simulink model "RCAMSimulation"  (R2024b)
settings: Solver=VariableStepAuto  StartTime=0.0  StopTime=TF  FixedStep=0.05  RelTol=1e-3
values from neighbouring files (symbols this model uses):
  u1max = deg2rad(25)    [RCAM_model.m]    (also in RCAM_model_navigation.m)
  u1min = deg2rad(-25)    [RCAM_model.m]    (also in RCAM_model_navigation.m)
  u2max = deg2rad(10)    [RCAM_model.m]    (also in RCAM_model_navigation.m)
  u2min = deg2rad(-25)    [RCAM_model.m]    (also in RCAM_model_navigation.m)
  u3max = deg2rad(30)    [RCAM_model.m]    (also in RCAM_model_navigation.m)
  u3min = deg2rad(-30)    [RCAM_model.m]    (also in RCAM_model_navigation.m)
  u4max = deg2rad(10)    [RCAM_model.m]    (also in RCAM_model_navigation.m)
  u4min = deg2rad(0.5)    [RCAM_model.m]    (also in RCAM_model_navigation.m)
  u5max = u4max    [RCAM_model.m]    (also in RCAM_model_navigation.m)
  u5min = u4min    [RCAM_model.m]    (also in RCAM_model_navigation.m)
  U_bar = Z_bar(10:14)    [RCAM_LQR_Trim.m]    (also in RCAM_LQR_Trim_navigation.m = Z_bar(13:17))
  X_bar = Z_bar(1:9)    [RCAM_LQR_Trim.m]    (also in RCAM_LQR_Trim_navigation.m)
undefined symbols (not defined in the file or in its folder): ail_dist, dist_dt, GEO0, K, navigation_from_state, P0, RB211, RCAM_model, rud_dist, stab_dist, x0
libraries: aerolibfltsims x2, vrlib x1, aerolibanimutils x1
settings Model: Creator=jaspergeldenbott  LastModifiedBy=jaspergeldenbott
settings RTWCC: GPUComputeCapability=3.5

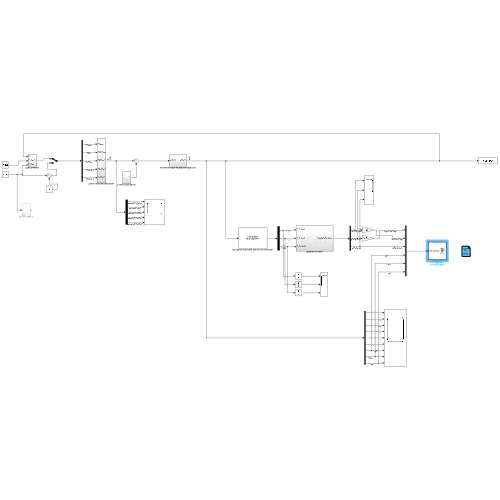
[thumbnail: Simulink's stored preview of the top-level diagram]
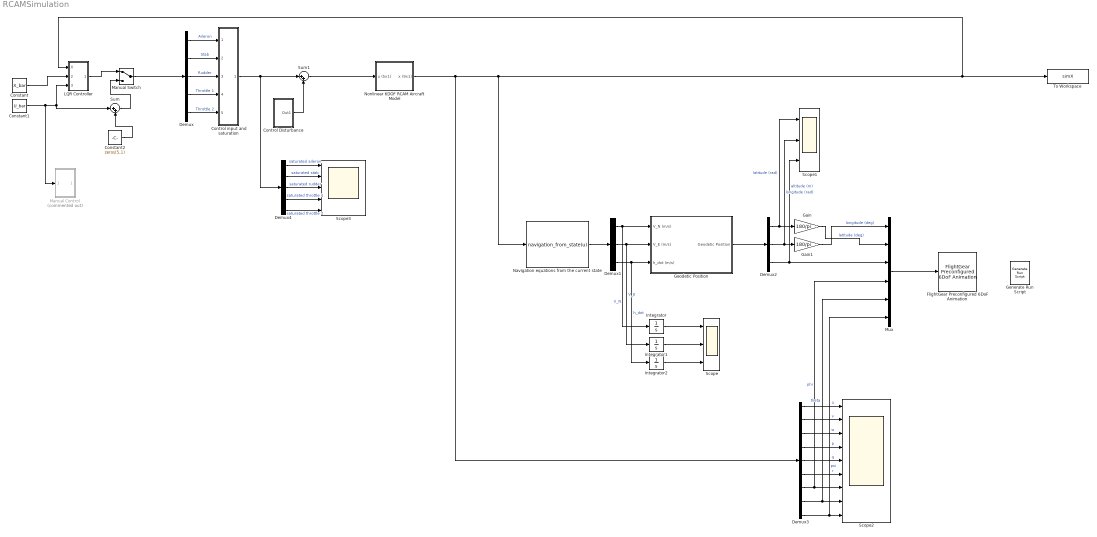
== system RCAMSimulation ==
  Constant : Constant  Value=X_bar
  Constant1 : Constant  Value=U_bar
  Constant2 : Constant  Value=zeros(5,1)
  Control Disturbance : Subsystem
  Control input and saturation : Subsystem
  Demux : Demux  Outputs=5
  Demux1 : Demux  Outputs=3
  Demux2 : Demux  Outputs=3
  Demux3 : Demux  Outputs=9
  Demux4 : Demux  Outputs=5
  FlightGear Preconfigured 6DoF Animation : aerolibfltsims/FlightGear Preconfigured 6DoF Animation  xFlightGearVersion=v2019.1  DestinationIpAddress=127.0.0.1  DestinationPort=5502  SampleTime=1/200  packetVersion=24
  Gain : Gain  Gain=180/pi
  Gain1 : Gain  Gain=180/pi
  Generate Run Script : aerolibfltsims/Generate Run Script  Architecture=Mac  dataFlow=Send  GeometryModelName=757-200-RB211  AirportId=KSFO  RunwayId=10L  InitialAltitude=7224  InitialHeading=113  OffsetDistance=4.72  OffsetAzimuth=0  InstallScenery=off  DisableShaders=off  OriginAddress=127.0.0.1  DestinationPort=5502  OriginPort=5505  LocalAddress=127.0.0.1  OutputFileName=runfg.bat  FlightGearBaseDirectory=/Applications/FlightGear.app
  Geodetic Position : Subsystem
  Integrator : Integrator  InitialCondition=P0(1)
  Integrator1 : Integrator  InitialCondition=P0(2)
  Integrator2 : Integrator  InitialCondition=P0(3)
  LQR Controller : Subsystem
  Manual Control : Subsystem  Commented=on
  Manual Switch : ManualSwitch
  Mux : Mux  Inputs=6
  Navigation equations from the current state : MATLABFcn  MATLABFcn=navigation_from_state(u)
  Nonlinear 6DOF RCAM Aircraft Model : Subsystem
  Scope : Scope  NumInputPorts=3
  Scope1 : Scope  NumInputPorts=3
  Scope2 : Scope  NumInputPorts=9
  Scope3 : Scope  NumInputPorts=5
  Sum : Sum  Inputs=|++
  Sum1 : Sum  Inputs=|++
  To Workspace : ToWorkspace  VariableName=simX  SaveFormat=Timeseries  SampleTime=-1
  wires:
  Nonlinear 6DOF RCAM Aircraft Model/1(x (9x1)) -> To Workspace/1, LQR Controller/1(X), Navigation equations from the current state/1, Demux3/1
  Demux/4 -> Control input and saturation/4(Throttle 1)  "Throttle 1"
  Demux/3 -> Control input and saturation/3(Rudder)  "Rudder"
  Demux/1 -> Control input and saturation/1(Aileron)  "Aileron"
  Demux/5 -> Control input and saturation/5(Trottle 2)  "Throttle 2"
  Demux/2 -> Control input and saturation/2(Stabilizer)  "Stab"
  Navigation equations from the current state/1 -> Demux1/1
  Demux1/1 -> Integrator/1, Geodetic Position/1(V_N (m/s))  "V_N"
  Demux1/2 -> Integrator1/1, Geodetic Position/2(V_E (m/s))  "V_E"
  Demux1/3 -> Integrator2/1, Geodetic Position/3(h_dot (m/s))  "h_dot"
  Integrator/1 -> Scope/1
  Integrator1/1 -> Scope/2
  Integrator2/1 -> Scope/3
  Geodetic Position/1(Geodetic Position) -> Demux2/1
  Demux2/1 -> Scope1/1, Gain/1  "latitude (rad)"
  Demux2/2 -> Scope1/2, Gain1/1  "longitude (rad)"
  Demux2/3 -> Scope1/3, Mux/3  "altitude (m)"
  Constant/1 -> LQR Controller/2(X_bar)
  Constant1/1 -> Manual Control/1(In1), LQR Controller/3(U_bar), Sum/1
  LQR Controller/1(Out1) -> Manual Switch/1
  Gain1/1 -> Mux/1  "longitude (deg)"
  Gain/1 -> Mux/2  "latitude (deg)"
  Mux/1 -> FlightGear Preconfigured 6DoF Animation/1
  Demux3/1 -> Scope2/1  "u"
  Demux3/2 -> Scope2/2  "v"
  Demux3/3 -> Scope2/3  "w"
  Demux3/4 -> Scope2/4  "p"
  Demux3/5 -> Scope2/5  "q"
  Demux3/6 -> Scope2/6  "r"
  Demux3/7 -> Mux/4, Scope2/7  "phi"
  Demux3/8 -> Mux/5, Scope2/8  "theta"
  Demux3/9 -> Mux/6, Scope2/9  "psi"
  Control Disturbance/1(Out1) -> Sum1/2
  Constant2/1 -> Sum/2
  Sum/1 -> Manual Switch/2
  Control input and saturation/1(Out1) -> Demux4/1, Sum1/1
  Sum1/1 -> Nonlinear 6DOF RCAM Aircraft Model/1(u (5x1))
  Manual Switch/1 -> Demux/1
  Demux4/1 -> Scope3/1  "saturated aileron"
  Demux4/2 -> Scope3/2  "saturated stab"
  Demux4/3 -> Scope3/3  "saturated rudder"
  Demux4/4 -> Scope3/4  "saturated throttle 1"
  Demux4/5 -> Scope3/5  "saturated throttle 2"

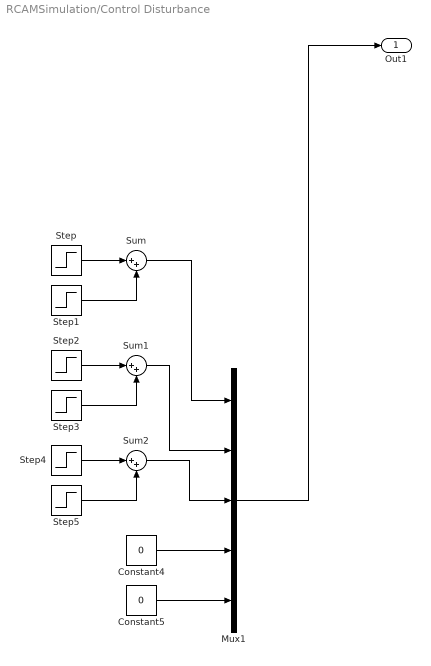
== system RCAMSimulation/Control Disturbance ==
  Constant4 : Constant  Value=0
  Constant5 : Constant  Value=0
  Mux1 : Mux  Inputs=5
  Step : Step  Time=10  After=ail_dist*pi/180  SampleTime=0
  Step1 : Step  Time=10 + dist_dt  After=-ail_dist*pi/180  SampleTime=0
  Step2 : Step  Time=10  After=stab_dist*pi/180  SampleTime=0
  Step3 : Step  Time=10 + dist_dt  After=-stab_dist*pi/180  SampleTime=0
  Step4 : Step  Time=10  After=rud_dist*pi/180  SampleTime=0
  Step5 : Step  Time=10 + dist_dt  After=-rud_dist*pi/180  SampleTime=0
  Sum : Sum  Inputs=|++
  Sum1 : Sum  Inputs=|++
  Sum2 : Sum  Inputs=|++
  Out1 : Outport
  wires:
  Sum/1 -> Mux1/1
  Constant5/1 -> Mux1/5
  Sum1/1 -> Mux1/2
  Step1/1 -> Sum/2
  Mux1/1 -> Out1/1
  Step/1 -> Sum/1
  Constant4/1 -> Mux1/4
  Step3/1 -> Sum1/2
  Step2/1 -> Sum1/1
  Step5/1 -> Sum2/2
  Step4/1 -> Sum2/1
  Sum2/1 -> Mux1/3

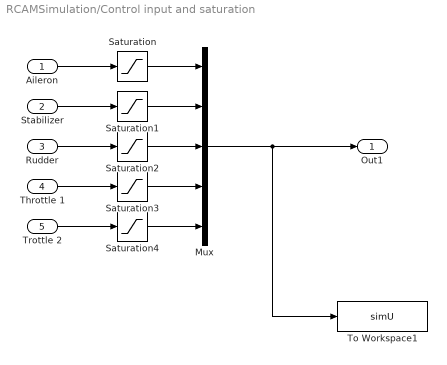
== system RCAMSimulation/Control input and saturation ==
  Aileron : Inport
  Stabilizer : Inport  Port=2
  Rudder : Inport  Port=3
  Throttle 1 : Inport  Port=4
  Trottle 2 : Inport  Port=5
  Mux : Mux  Inputs=5
  Saturation : Saturate  UpperLimit=u1max  LowerLimit=u1min
  Saturation1 : Saturate  UpperLimit=u2max  LowerLimit=u2min
  Saturation2 : Saturate  UpperLimit=u3max  LowerLimit=u3min
  Saturation3 : Saturate  UpperLimit=u4max  LowerLimit=u4min
  Saturation4 : Saturate  UpperLimit=u5max  LowerLimit=u5min
  To Workspace1 : ToWorkspace  VariableName=simU  SaveFormat=Timeseries  SampleTime=-1
      settings: MaxDataPoints=100000
  Out1 : Outport
  wires:
  Mux/1 -> To Workspace1/1, Out1/1
  Aileron/1 -> Saturation/1
  Saturation/1 -> Mux/1
  Stabilizer/1 -> Saturation1/1
  Saturation1/1 -> Mux/2
  Rudder/1 -> Saturation2/1
  Saturation2/1 -> Mux/3
  Throttle 1/1 -> Saturation3/1
  Saturation3/1 -> Mux/4
  Trottle 2/1 -> Saturation4/1
  Saturation4/1 -> Mux/5

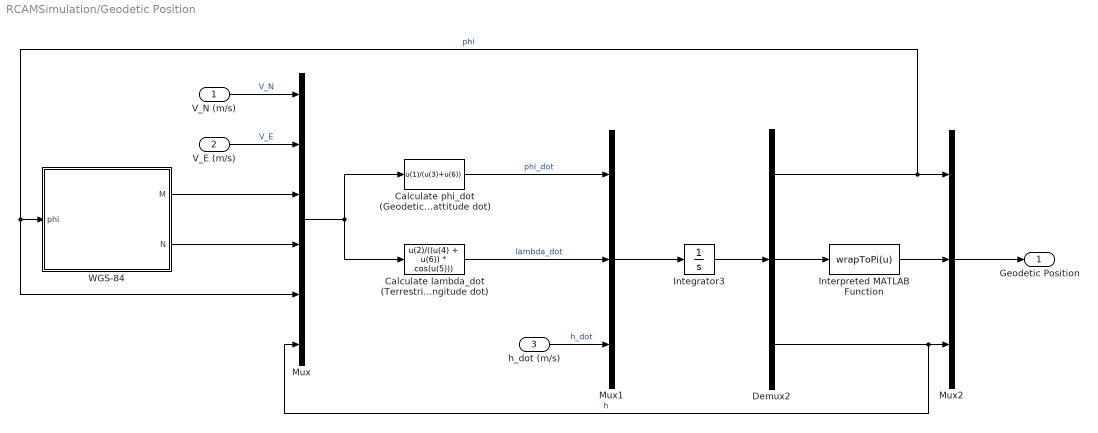
== system RCAMSimulation/Geodetic Position ==
  V_N (m/s) : Inport
  V_E (m/s) : Inport  Port=2
  h_dot (m/s) : Inport  Port=3
  Calculate lambda_dot (Terrestrial Longitude dot) : Fcn  Expr=u(2)/((u(4) + u(6)) * cos(u(5)))
  Calculate phi_dot (Geodetic Lattitude dot) : Fcn  Expr=u(1)/(u(3)+u(6))
  Demux2 : Demux  Outputs=3
  Integrator3 : Integrator  InitialCondition=GEO0
  Interpreted MATLAB Function : MATLABFcn  MATLABFcn=wrapToPi(u)
  Mux : Mux  Inputs=6
  Mux1 : Mux  Inputs=3
  Mux2 : Mux  Inputs=3
  WGS-84 : Subsystem
  Geodetic Position : Outport
  wires:
  V_N (m/s)/1 -> Mux/1  "V_N"
  V_E (m/s)/1 -> Mux/2  "V_E"
  WGS-84/2(N) -> Mux/4
  Demux2/3 -> Mux/6, Mux2/3  "h"
  Interpreted MATLAB Function/1 -> Mux2/2
  Calculate lambda_dot (Terrestrial Longitude dot)/1 -> Mux1/2  "lambda_dot"
  Mux2/1 -> Geodetic Position/1
  Demux2/2 -> Interpreted MATLAB Function/1
  h_dot (m/s)/1 -> Mux1/3  "h_dot"
  Mux/1 -> Calculate lambda_dot (Terrestrial Longitude dot)/1, Calculate phi_dot (Geodetic Lattitude dot)/1
  Mux1/1 -> Integrator3/1
  Calculate phi_dot (Geodetic Lattitude dot)/1 -> Mux1/1  "phi_dot"
  WGS-84/1(M) -> Mux/3
  Demux2/1 -> Mux/5, WGS-84/1(phi), Mux2/1  "phi"
  Integrator3/1 -> Demux2/1

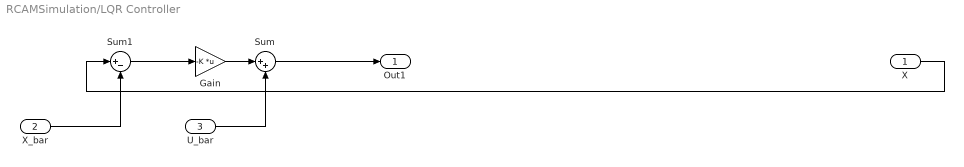
== system RCAMSimulation/LQR Controller ==
  X : Inport
  X_bar : Inport  Port=2
  U_bar : Inport  Port=3
  Gain : Gain  Gain=-K  Multiplication=Matrix(K*u)
  Sum : Sum  Inputs=|++
  Sum1 : Sum  Inputs=|+-
  Out1 : Outport
  wires:
  Gain/1 -> Sum/1
  X/1 -> Sum1/1
  Sum1/1 -> Gain/1
  Sum/1 -> Out1/1
  X_bar/1 -> Sum1/2
  U_bar/1 -> Sum/2

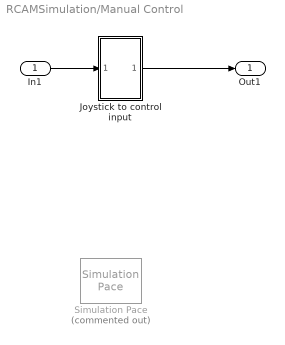
== system RCAMSimulation/Manual Control ==
  In1 : Inport
  Joystick to control input : Subsystem
  Simulation Pace : aerolibanimutils/Simulation Pace  Commented=on  SimulationPace=1  SleepMode=Auto  OutputPaceError=off  SampleTime=1/50
  Out1 : Outport
  wires:
  In1/1 -> Joystick to control input/1(U_bar)
  Joystick to control input/1(Out1) -> Out1/1

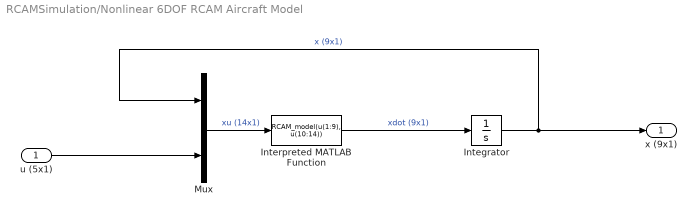
== system RCAMSimulation/Nonlinear 6DOF RCAM Aircraft Model ==
  u (5x1) : Inport
  Integrator : Integrator  InitialCondition=x0
  Interpreted MATLAB Function : MATLABFcn  MATLABFcn=RCAM_model(u(1:9), u(10:14))
  Mux : Mux  Inputs=2
  x (9x1) : Outport
  wires:
  u (5x1)/1 -> Mux/2
  Interpreted MATLAB Function/1 -> Integrator/1  "xdot (9x1)"
  Mux/1 -> Interpreted MATLAB Function/1  "xu (14x1)"
  Integrator/1 -> x (9x1)/1, Mux/1  "x (9x1)"

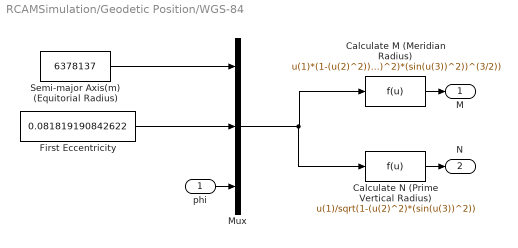
== system RCAMSimulation/Geodetic Position/WGS-84 ==
  phi : Inport
  Calculate M (Meridian Radius) : Fcn  Expr=u(1)*(1-(u(2)^2))/((1-(u(2)^2)*(sin(u(3))^2))^(3/2))
  Calculate N (Prime Vertical Radius) : Fcn  Expr=u(1)/sqrt(1-(u(2)^2)*(sin(u(3))^2))
  First Eccentricity : Constant  Value=0.081819190842622
  Mux : Mux  Inputs=3
  Semi-major Axis(m) (Equitorial Radius) : Constant  Value=6378137
  M : Outport
  N : Outport  Port=2
  wires:
  First Eccentricity/1 -> Mux/2
  phi/1 -> Mux/3
  Semi-major Axis(m) (Equitorial Radius)/1 -> Mux/1
  Calculate M (Meridian Radius)/1 -> M/1
  Calculate N (Prime Vertical Radius)/1 -> N/1
  Mux/1 -> Calculate N (Prime Vertical Radius)/1, Calculate M (Meridian Radius)/1

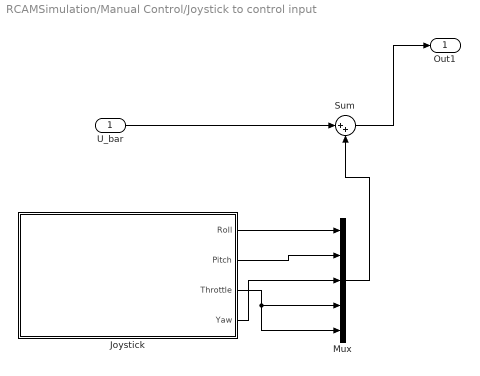
== system RCAMSimulation/Manual Control/Joystick to control input ==
  U_bar : Inport
  Joystick : Subsystem
  Mux : Mux  Inputs=5
  Sum : Sum  Inputs=|++
  Out1 : Outport
  wires:
  Sum/1 -> Out1/1
  Joystick/1(Roll) -> Mux/1
  Mux/1 -> Sum/2
  Joystick/3(Throttle) -> Mux/5, Mux/4
  Joystick/4(Yaw) -> Mux/3
  Joystick/2(Pitch) -> Mux/2
  U_bar/1 -> Sum/1

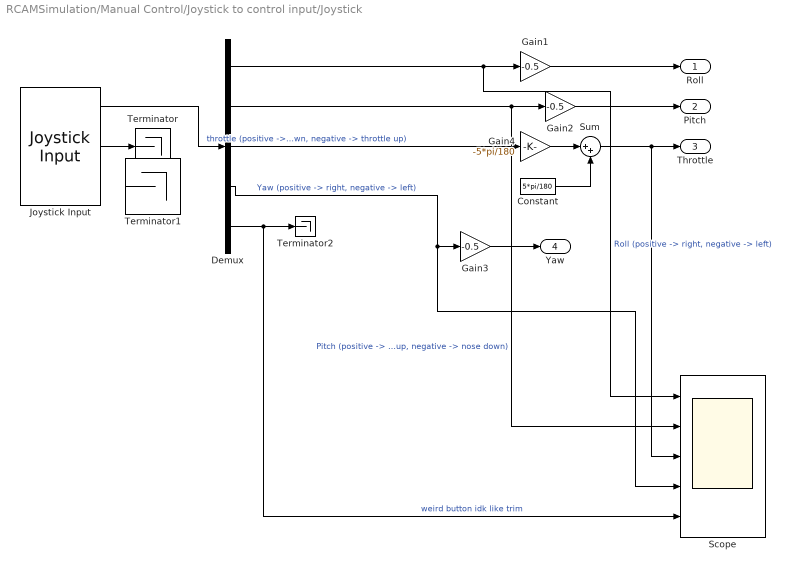
== system RCAMSimulation/Manual Control/Joystick to control input/Joystick ==
  Constant : Constant  Value=5*pi/180
  Demux : Demux  Outputs=5
  Gain1 : Gain  Gain=-0.5
  Gain2 : Gain  Gain=-0.5
  Gain3 : Gain  Gain=-0.5
  Gain4 : Gain  Gain=-5*pi/180
  Joystick Input : vrlib/Joystick Input  joyid=0  adjustports=on  forcefeed=off
  Scope : Scope  NumInputPorts=5
  Sum : Sum  Inputs=|++
  Terminator : Terminator
  Terminator1 : Terminator
  Terminator2 : Terminator
  Roll : Outport
  Pitch : Outport  Port=2
  Throttle : Outport  Port=3
  Yaw : Outport  Port=4
  wires:
  Demux/4 -> Scope/4, Gain3/1  "Yaw (positive -> right, negative -> left)"
  Demux/2 -> Scope/2, Gain2/1  "Pitch (positive -> nose up, negative -> nose down)"
  ? -> Terminator1/1
  Demux/3 -> Gain4/1  "throttle (positive -> throttle down, negative -> throttle up)"
  Joystick Input/1 -> Demux/1
  Joystick Input/2 -> Terminator/1
  Demux/1 -> Gain1/1, Scope/1  "Roll (positive -> right, negative -> left)"
  Demux/5 -> Terminator2/1, Scope/5  "weird button idk like trim"
  Constant/1 -> Sum/2
  Gain1/1 -> Roll/1
  Gain2/1 -> Pitch/1
  Gain3/1 -> Yaw/1
  Sum/1 -> Scope/3, Throttle/1
  Gain4/1 -> Sum/1
